simulink model "Main"  (R2022b)
settings: Solver=VariableStepAuto  StartTime=0.0  StopTime=10.0  RelTol=1e-3
settings Model: Creator=ASUS  LastModifiedBy=ASUS

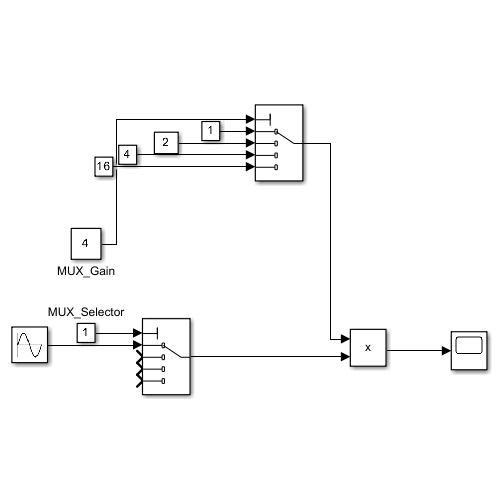
[thumbnail: Simulink's stored preview of the top-level diagram]
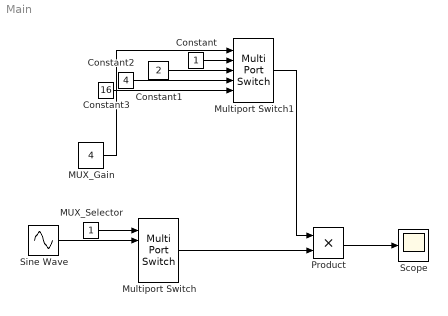
== system Main ==
  Constant : Constant
  Constant1 : Constant  Value=2
  Constant2 : Constant  Value=4
  Constant3 : Constant  Value=16
  MUX_Gain : Constant  Value=4
  MUX_Selector : Constant
  Multiport Switch : MultiPortSwitch  Inputs=4  SaturateOnIntegerOverflow=off  InputSameDT=off
  Multiport Switch1 : MultiPortSwitch  Inputs=4  SaturateOnIntegerOverflow=off  InputSameDT=off
  Product : Product
  Scope : Scope
  Sine Wave : Sin  SampleTime=0
  wires:
  MUX_Selector/1 -> Multiport Switch/1
  Multiport Switch/1 -> Product/2
  MUX_Gain/1 -> Multiport Switch1/1
  Constant/1 -> Multiport Switch1/2
  Constant1/1 -> Multiport Switch1/3
  Constant2/1 -> Multiport Switch1/4
  Constant3/1 -> Multiport Switch1/5
  Multiport Switch1/1 -> Product/1
  Product/1 -> Scope/1
  Sine Wave/1 -> Multiport Switch/2
